simulink model "questao3"  (R2015b)
settings: Solver=VariableStepAuto  StartTime=0.0  StopTime=0.01  RelTol=1e-3
libraries: dsparch4 x1
settings Model: Creator=Aluno  LastModifiedBy=Aluno

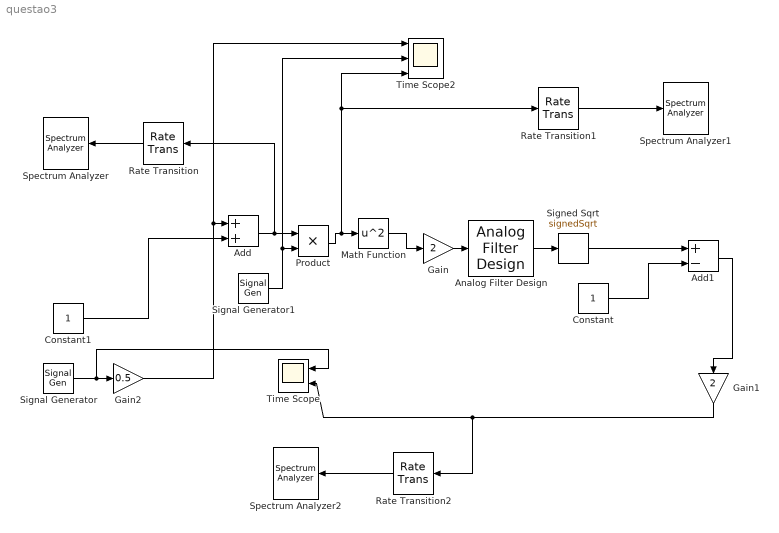
== system questao3 ==
  Add : Sum
  Add1 : Sum  Inputs=+-
  Analog Filter Design : dsparch4/Analog Filter Design  method=Butterworth  filttype=Lowpass  N=8  Wlo=2*pi  Whi=80  Rp=2  Rs=40
  Constant : Constant
  Constant1 : Constant
  Gain : Gain  Gain=2
  Gain1 : Gain  Gain=2
  Gain2 : Gain  Gain=0.5
  Math Function : Math  Operator=square  SaturateOnIntegerOverflow=on
  Product : Product
  Rate Transition : RateTransition
  Rate Transition1 : RateTransition
  Rate Transition2 : RateTransition
  Signal Generator : SignalGenerator  Frequency=1000
  Signal Generator1 : SignalGenerator  Frequency=20000
  Signed Sqrt : Sqrt  Operator=signedSqrt  SaturateOnIntegerOverflow=on
  Spectrum Analyzer : SpectrumAnalyzer
  Spectrum Analyzer1 : SpectrumAnalyzer
  Spectrum Analyzer2 : SpectrumAnalyzer
  Time Scope : Scope  NumInputPorts=2
  Time Scope2 : Scope  NumInputPorts=3
  wires:
  Constant1/1 -> Add/2
  Rate Transition1/1 -> Spectrum Analyzer1/1
  Add/1 -> Rate Transition/1, Product/1
  Product/1 -> Rate Transition1/1, Time Scope2/3, Math Function/1
  Math Function/1 -> Gain/1
  Gain/1 -> Analog Filter Design/1
  Rate Transition/1 -> Spectrum Analyzer/1
  Rate Transition2/1 -> Spectrum Analyzer2/1
  Gain1/1 -> Rate Transition2/1, Time Scope/2
  Add1/1 -> Gain1/1
  Constant/1 -> Add1/2
  Signed Sqrt/1 -> Add1/1
  Analog Filter Design/1 -> Signed Sqrt/1
  Signal Generator/1 -> Time Scope/1, Gain2/1
  Gain2/1 -> Add/1, Time Scope2/1
  Signal Generator1/1 -> Time Scope2/2, Product/2
